simulink model "Harness_EXV_OpenLoop"  (R2025b)
settings: Solver=VariableStepAuto  StartTime=0.0  StopTime=10.0  RelTol=1e-3
undefined symbols (not defined in the file): A_min, opening_cmd
libraries: fl_lib x4, nesl_utility x3, SimscapeFluids_lib x1
settings Model: Creator=altoa  LastModifiedBy=altoa

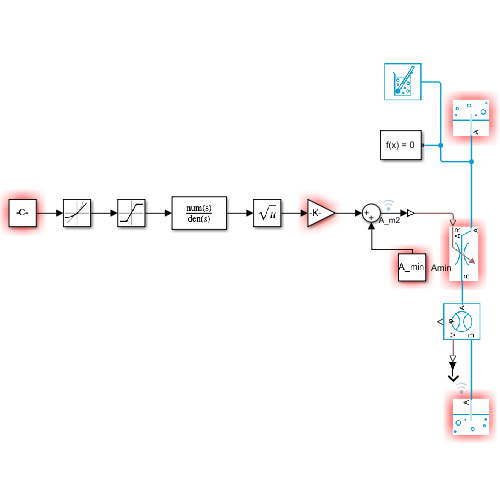
[thumbnail: Simulink's stored preview of the top-level diagram]
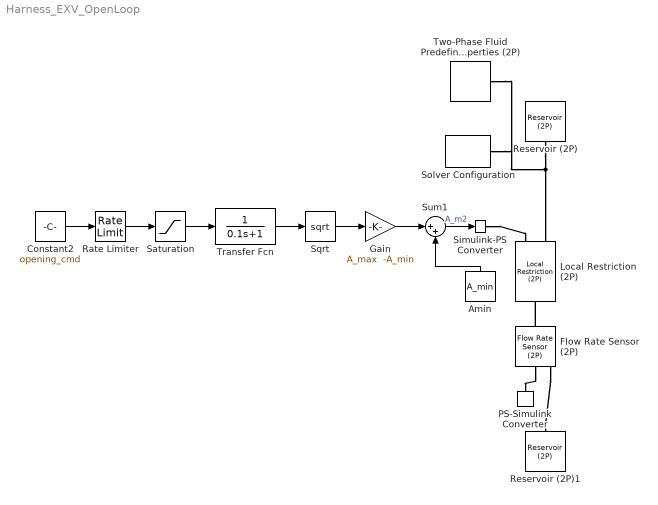
== system Harness_EXV_OpenLoop ==
  Amin : Constant  Value=A_min  VectorParams1D=off
  Constant2 : Constant  Value=opening_cmd
  Flow Rate Sensor (2P) : fl_lib/Two-Phase Fluid/Sensors/Flow Rate Sensor (2P)  mass_flow_measure=true  volumetric_flow_measure=false  energy_flow_measure=true
      settings: InternalSimscapePortConfiguration="{\"Bottom\":[{\"id\":\"PHI\",\"label\":\"φ\",\"type\":\"output\"}],\"Left\":[{\"id\":\"A\",\"label\":\"A\",\"type\":\"foundation.two_phase_fluid.two_phase_fluid\"}],\"Right\":[{\"id\":\"B\",\"label\":\"B\",\"type\":\"foundation.two_phase_fluid.two_phase_fluid\"},{\"id\":\"M\",\"label\":\"M\",\"type\":\"output\"}],\"Top\":[]}"
  Gain : Gain  Gain="A_max  -A_min"
  Local Restriction (2P) : fl_lib/Two-Phase Fluid/Elements/Local Restriction (2P)  restriction_type=foundation.enum.restriction_type.variable  restriction_area=1e-3 m^2  min_area=A_min m^2  max_area=A_max m^2  pressure_loss_model=foundation.enum.RestrictionPressureLossModel.Bernoulli  area=pi*0.02^2/4 m^2  Cd=0.64  B_lam=0.999
      settings: InternalSimscapePortConfiguration="{\"Bottom\":[],\"Left\":[{\"id\":\"A\",\"label\":\"A\",\"type\":\"foundation.two_phase_fluid.two_phase_fluid\"},{\"id\":\"area_in\",\"label\":\"AR\",\"type\":\"input\"}],\"Right\":[{\"id\":\"B\",\"label\":\"B\",\"type\":\"foundation.two_phase_fluid.two_phase_fluid\"}],\"Top\":[]}"
  PS-Simulink Converter : nesl_utility/PS-Simulink Converter  PhysicalDomain=network_engine_domain  SubClassName=ps_output  LeftPortType=input  RightPortType=output  PseudoPeriodic=off  Frequencies=[]  VectorFormat=inherit  Unit=inherit  AffineConversion=off
  Rate Limiter : RateLimiter  RisingSlewLimit=0.03  FallingSlewLimit=- 0.03  SampleTimeMode=inherited  LinearizeAsGain=off
  Reservoir (2P) : fl_lib/Two-Phase Fluid/Elements/Reservoir (2P)  pressure_spec=foundation.enum.ReservoirPressureSpec2P.Specified  reservoir_pressure="p_high_set  Pa"  reservoir_condensing_temperature=373.15 K  reservoir_evaporating_temperature=373.15 K  energy_spec=foundation.enum.ReservoirEnergySpec2P.Temperature  reservoir_temperature=38 degC  reservoir_quality=0.5  reservoir_void_fraction=0.5  reservoir_enthalpy=1500 kJ/kg  reservoir_internal_energy=1500 kJ/kg  reservoir_subcooling=5 deltaK  reservoir_superheating=5 deltaK  area_A=0.01 m^2
  Reservoir (2P)1 : fl_lib/Two-Phase Fluid/Elements/Reservoir (2P)  pressure_spec=foundation.enum.ReservoirPressureSpec2P.Specified  reservoir_pressure=p_low_set Pa  reservoir_condensing_temperature=373.15 K  reservoir_evaporating_temperature=373.15 K  energy_spec=foundation.enum.ReservoirEnergySpec2P.Temperature  reservoir_temperature=temp_low_set degC  reservoir_quality=0.5  reservoir_void_fraction=0.5  reservoir_enthalpy=1500 kJ/kg  reservoir_internal_energy=1500 kJ/kg  reservoir_subcooling=5 deltaK  reservoir_superheating=5 deltaK  area_A=0.01 m^2
  Saturation : Saturate  UpperLimit=1  LowerLimit=0
  Simulink-PS Converter : nesl_utility/Simulink-PS Converter  PhysicalDomain=network_engine_domain  SubClassName=ps_input  LeftPortType=input  RightPortType=output  PseudoPeriodic=off  Frequencies=[]  NoiseDistribution=none  NoiseParameters=[]  Unit=m^2  AffineConversion=off  FilteringAndDerivatives=provide  SimscapeFilterOrder=1  InputFilterTimeConstant=0.001  UdotUserProvided=0
  Solver Configuration : nesl_utility/Solver Configuration  PhysicalDomain=network_engine_domain  SubClassName=solver  LeftPortType=input  RightPortType=generic  Tones=[]  Harmonics=[]  SimulateNoise=off  Profile=off  UseLocalSampling=off  EnableSwitchedLinearOptims=on  FrequencyDomain=off  UseCCode=off  RelTol=0.001  AbsTol=0.001  MinStep=1e-09  ToWorkspace=off  RevertToSquareIcSolve=off  NumHomotopyIterations=100  PhasorMode=off  PhasorModeNumHarmonics=1  ConsistencySolver=NEWTON_XTOL_AFTER_FTOL  IndexReductionMethod=DerivativeReplacement  DoDC=off  ResidualTolerance=1e-09  ConsistencyTolSource=GLOBAL  ConsistencyAbsTol=0.001  ConsistencyRelTol=0.001  ConsistencyTolFactor=0.001  UseLocalSolver=off  LocalSolverChoice=NE_BACKWARD_EULER_ADVANCER  ResolveIndetEquations=on  FunctionEvalNumThread=1  LocalSolverSampleTime=0.001  DoFixedCost=off  MaxNonlinIter=3  MaxModeIter=2  ComputeImpulses=off  ImpulseIterations=2  LinearAlgebra=auto  LinearAlgebraNumThread=0  EquationFormulation=NE_TIME_EF  DelaysMemoryBudget=1024  AutomaticFiltering=on  FilteringTimeConstant=0.001  PartitionStorageMethod=AS_NEEDED  PartitionMemoryBudget=1024  PartitionMethod=ROBUST  MultibodyUseLocalSolver=off  MultibodyLocalSolverChoice=ODE1  MultibodyLocalSolverSampleTime=0.001
  Sqrt : Sqrt
  Sum1 : Sum  Inputs=|++
  Transfer Fcn : TransferFcn  Numerator=1  Denominator="[0.1  1]"
  Two-Phase Fluid Predefined Properties (2P) : SimscapeFluids_lib/Two-Phase Fluid/Utilities/Two-Phase Fluid Predefined Properties (2P)  fluid=fluids.two_phase_fluid.utilities.enum.Fluid.R32  p_atm=0.101325 MPa  properties_range_check=simscape.enum.assert.action.error  q_rev=0.01 Pa
  wires:
  Amin/1 -> Sum1/2
  Sum1/1 -> Simulink-PS Converter/1  "A_m2"
  Transfer Fcn/1 -> Sqrt/1
  Saturation/1 -> Transfer Fcn/1
  Sqrt/1 -> Gain/1
  Rate Limiter/1 -> Saturation/1
  Constant2/1 -> Rate Limiter/1
  Gain/1 -> Sum1/1
  connections:
  Simulink-PS Converter/RConn1 -- Local Restriction (2P)/LConn2
  Reservoir (2P)/LConn1 -- Two-Phase Fluid Predefined Properties (2P)/RConn1 -- Solver Configuration/RConn1 -- Local Restriction (2P)/LConn1
  Flow Rate Sensor (2P)/RConn1 -- Reservoir (2P)1/LConn1
  Flow Rate Sensor (2P)/LConn1 -- Local Restriction (2P)/RConn1
  Flow Rate Sensor (2P)/RConn2 -- PS-Simulink Converter/LConn1
